simulink model "InportDimensions"  (R2017b)
settings: Solver=FixedStepDiscrete  StartTime=0.0  StopTime=10.0  FixedStep=0.200000  RelTol=1e-3
settings Model: Creator=hbourbou  LastModifiedBy=hbourbou
settings DataIOCC: SaveFormat=StructureWithTime
settings OptimizationCC: LifeSpan=inf
settings DebuggingCC: SFExecutionAtInitializationDiag=none
settings HardwareCC: ProdBitPerSizeT=32  ProdBitPerPtrDiffT=32  ProdWordSize=32  ProdHWDeviceType=Specified
settings CodeAppCC: StateflowObjectComments=on

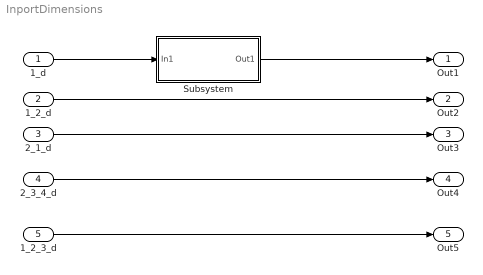
== system InportDimensions ==
  1_d : Inport
  1_2_d : Inport  Port=2  OutDataTypeStr=double  PortDimensions=[1 2]
  2_1_d : Inport  Port=3  PortDimensions=[2 1]
  2_3_4_d : Inport  Port=4  PortDimensions=[2 3 4]
  1_2_3_d : Inport  Port=5  PortDimensions=[1 2 3]
  Subsystem : Subsystem
  Out1 : Outport  OutMin=1  OutMax=5
  Out2 : Outport  Port=2
  Out3 : Outport  Port=3
  Out4 : Outport  Port=4
  Out5 : Outport  Port=5
  wires:
  1_d/1 -> Subsystem/1(In1)
  1_2_d/1 -> Out2/1
  2_1_d/1 -> Out3/1
  2_3_4_d/1 -> Out4/1
  1_2_3_d/1 -> Out5/1
  Subsystem/1(Out1) -> Out1/1

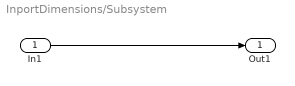
== system InportDimensions/Subsystem ==
  In1 : Inport
  Out1 : Outport
  wires:
  In1/1 -> Out1/1
